simulink model "PS_top"  (R2020b)
settings: Solver=VariableStepAuto  StartTime=0.0  StopTime=10.0  RelTol=1e-3
settings Model: DataDictionary=PS_top.sldd  Creator=ravenst1  LastModifiedBy=ravenst1

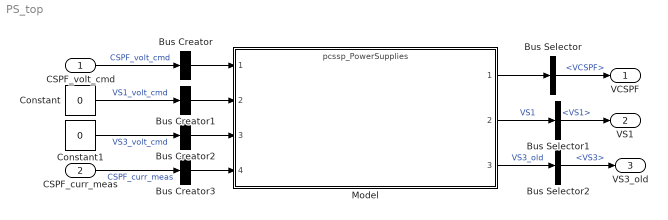
== system PS_top ==
  CSPF_volt_cmd : Inport
  CSPF_curr_meas : Inport  Port=2
  Bus Creator : BusCreator  Inputs=1  OutDataTypeStr=Bus: pcssp_PS_CSPF_volt_cmd
  Bus Creator1 : BusCreator  Inputs=1  OutDataTypeStr=Bus: pcssp_PS_VS1_volt_cmd
  Bus Creator2 : BusCreator  Inputs=1  OutDataTypeStr=Bus: pcssp_PS_VS3_volt_cmd
  Bus Creator3 : BusCreator  Inputs=1  OutDataTypeStr=Bus: pcssp_PS_CSPF_curr_meas
  Bus Selector : BusSelector  OutputSignals=VCSPF
  Bus Selector1 : BusSelector  OutputSignals=VS1
  Bus Selector2 : BusSelector  OutputSignals=VS3
  Constant : Constant  Value=0
  Constant1 : Constant  Value=0
  Model : ModelReference  ModelNameDialog=pcssp_PowerSupplies.slx  UsingDefaultArgumentValue=0  SimulationMode=Normal  ModelReferenceVersion=1.37
  VCSPF : Outport
  VS1 : Outport  Port=2
  VS3_old : Outport  Port=3
  wires:
  CSPF_volt_cmd/1 -> Bus Creator/1  "CSPF_volt_cmd"
  Bus Creator/1 -> Model/1
  CSPF_curr_meas/1 -> Bus Creator3/1  "CSPF_curr_meas"
  Bus Creator3/1 -> Model/4
  Bus Creator2/1 -> Model/3
  Constant1/1 -> Bus Creator2/1  "VS3_volt_cmd"
  Constant/1 -> Bus Creator1/1  "VS1_volt_cmd"
  Bus Creator1/1 -> Model/2
  Model/1 -> Bus Selector/1
  Bus Selector/1 -> VCSPF/1  "<VCSPF>"
  Model/2 -> Bus Selector1/1  "VS1"
  Bus Selector1/1 -> VS1/1  "<VS1>"
  Model/3 -> Bus Selector2/1  "VS3_old"
  Bus Selector2/1 -> VS3_old/1  "<VS3>"
